simulink model "carestimation_calculation"  (Simulink 8.1)
settings: Solver=ode45  StartTime=0.0  StopTime=10.0  RelTol=1e-3
libraries: simulink x2, simulink_extras x1
settings Model: Creator=eric  LastModifiedBy=eric
settings DataIOCC: SignalLoggingSaveFormat=Dataset
settings OptimizationCC: ExpressionDepthLimit=128
settings DebuggingCC: FcnCallInpInsideContextMsg=EnableAllAsError
settings GRTTargetCC: CombineOutputUpdateFcns=on  GRTInterface=off

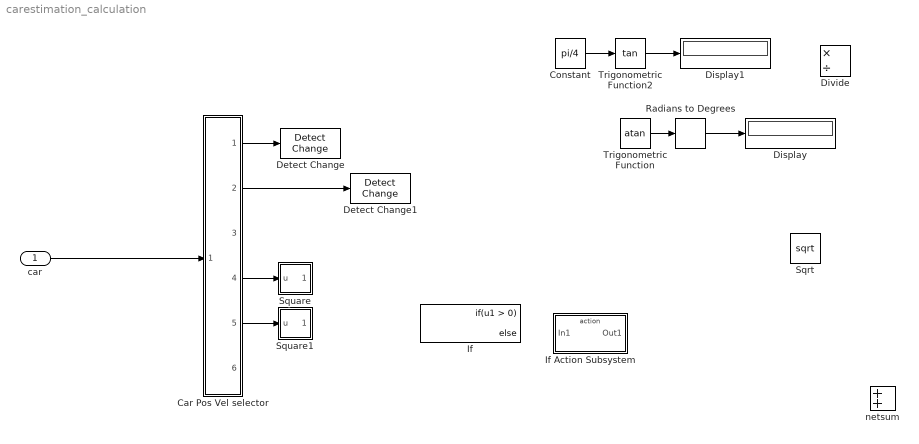
== system carestimation_calculation ==
  car : Inport
  Car Pos Vel selector : Subsystem
  Constant : Constant  Value=pi/4
  Detect Change : simulink/Logic and Bit Operations/Detect Change  vinit=0  InputProcessing=Inherited  OutDataTypeStr=boolean
  Detect Change1 : simulink/Logic and Bit Operations/Detect Change  vinit=0  InputProcessing=Inherited  OutDataTypeStr=boolean
  Display : Display
  Display1 : Display
  Divide : Product  Inputs=*/
  If : If
  If Action Subsystem : Subsystem  TreatAsAtomicUnit=on
  Radians to Degrees : simulink_extras/Transformations/Radians to Degrees
  Sqrt : Sqrt  SaturateOnIntegerOverflow=on
  Square : Subsystem
  Square1 : Subsystem
  Trigonometric Function : Trigonometry  Operator=atan
  Trigonometric Function2 : Trigonometry  Operator=tan
  netsum : Sum  Inputs=2  SaturateOnIntegerOverflow=on  InputSameDT=on  OutDataTypeStr=Inherit: Same as first input
  wires:
  car/1 -> Car Pos Vel selector/1(car)
  Trigonometric Function2/1 -> Display1/1
  Constant/1 -> Trigonometric Function2/1
  Trigonometric Function/1 -> Radians to Degrees/1
  Radians to Degrees/1 -> Display/1
  Car Pos Vel selector/4(VX) -> Square/1(u)
  Car Pos Vel selector/5(VY) -> Square1/1(u)
  Car Pos Vel selector/1(PX) -> Detect Change/1
  Car Pos Vel selector/2(PY) -> Detect Change1/1

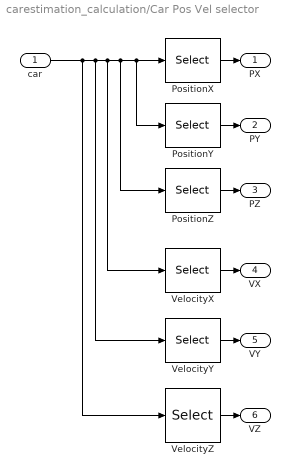
== system carestimation_calculation/Car Pos Vel selector ==
  car : Inport
  PositionX : Selector  InputPortWidth=12  IndexOptions=Index vector (dialog)  Indices=1  OutputSizes=1
  PositionY : Selector  InputPortWidth=12  IndexOptions=Index vector (dialog)  Indices=2  OutputSizes=1
  PositionZ : Selector  InputPortWidth=12  IndexOptions=Index vector (dialog)  Indices=3  OutputSizes=1
  VelocityX : Selector  InputPortWidth=12  IndexOptions=Index vector (dialog)  Indices=7  OutputSizes=1
  VelocityY : Selector  InputPortWidth=12  IndexOptions=Index vector (dialog)  Indices=8  OutputSizes=1
  VelocityZ : Selector  InputPortWidth=12  IndexOptions=Index vector (dialog)  Indices=9  OutputSizes=1
  PX : Outport
  PY : Outport  Port=2
  PZ : Outport  Port=3
  VX : Outport  Port=4
  VY : Outport  Port=5
  VZ : Outport  Port=6
  wires:
  VelocityZ/1 -> VZ/1
  car/1 -> VelocityZ/1, VelocityY/1, VelocityX/1, PositionZ/1, PositionY/1, PositionX/1
  PositionX/1 -> PX/1
  PositionY/1 -> PY/1
  VelocityX/1 -> VX/1
  PositionZ/1 -> PZ/1
  VelocityY/1 -> VY/1

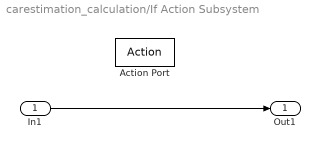
== system carestimation_calculation/If Action Subsystem ==
  In1 : Inport
  Action Port : ActionPort
  Out1 : Outport
  wires:
  In1/1 -> Out1/1

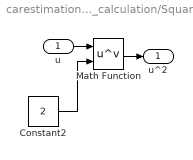
== system carestimation_calculation/Square ==
  u : Inport
  Constant2 : Constant  Value=2
  Math Function : Math  Operator=pow  SaturateOnIntegerOverflow=on
  u^2 : Outport
  wires:
  Constant2/1 -> Math Function/2
  Math Function/1 -> u^2/1
  u/1 -> Math Function/1

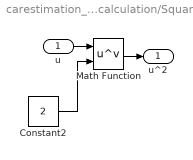
== system carestimation_calculation/Square1 ==
  u : Inport
  Constant2 : Constant  Value=2
  Math Function : Math  Operator=pow  SaturateOnIntegerOverflow=on
  u^2 : Outport
  wires:
  Constant2/1 -> Math Function/2
  Math Function/1 -> u^2/1
  u/1 -> Math Function/1
